simulink model "Pulse_Block"  (R2013b)
settings: Solver=ode3  StartTime=0.0  StopTime=2e-3  FixedStep=sampleTime  MaxStep=MaxStepSize  RelTol=1e-3
undefined symbols (not defined in the file or in its folder): Low, periSam
libraries: dspswit3 x4, simulink x2
settings Model: ExtModeTrigDuration=100  Creator=mainster  LastModifiedBy=mainster
settings OptimizationCC: OptimizeModelRefInitCode=on  LifeSpan=1
settings DebuggingCC: SolverPrmCheckMsg=none
settings HardwareCC: ProdLargestAtomicInteger=Long  ProdLargestAtomicFloat=Double  ProdEndianess=LittleEndian  ProdHWDeviceType=ARM Compatible->ARM Cortex
settings RTWCC: SystemTargetFile=realtime.tlc  GenerateMakefile=off  TemplateMakefile=realtime.tmf  Description=Run on Target Hardware  RTWVerbose=off  ProcessScript=realtime_make_rtw_hook
settings STFCustomTargetCC: TargetLibSuffix=.a  GenerateSampleERTMain=on  ERTCustomFileBanners=on  SupportNonInlinedSFcns=off  SupportVariableSizeSignals=on  MATLABClassNameForMDSCustomization=Simulink.SoftwareTarget.ERTCustomization  GRTInterface=off  SystemTargetFile=realtime.tlc
settings ERTTargetCC: CodeReplacementLibrary=ANSI_C  GenerateSampleERTMain=on  ParMdlRefBuildCompliant=off  CompOptLevelCompliant=off  ConcurrentExecutionCompliant=off  CombineOutputUpdateFcns=off  ERTFirstTimeCompliant=off  SupportContinuousTime=on  SupportVariableSizeSignals=on  ModelStepFunctionPrototypeControlCompliant=off  CPPClassGenCompliant=off  ExtModeMexArgs='192.168.2.111' 0 17725  InlinedParameterPlacement=NonHierarchical  ERTSrcFileBannerTemplate=realtime_code_template.cgt  ERTHdrFileBannerTemplate=realtime_code_template.cgt  ERTDataSrcFileTemplate=realtime_code_template.cgt  ERTDataHdrFileTemplate=realtime_code_template.cgt  ERTCustomFileTemplate=realtime_file_process.tlc

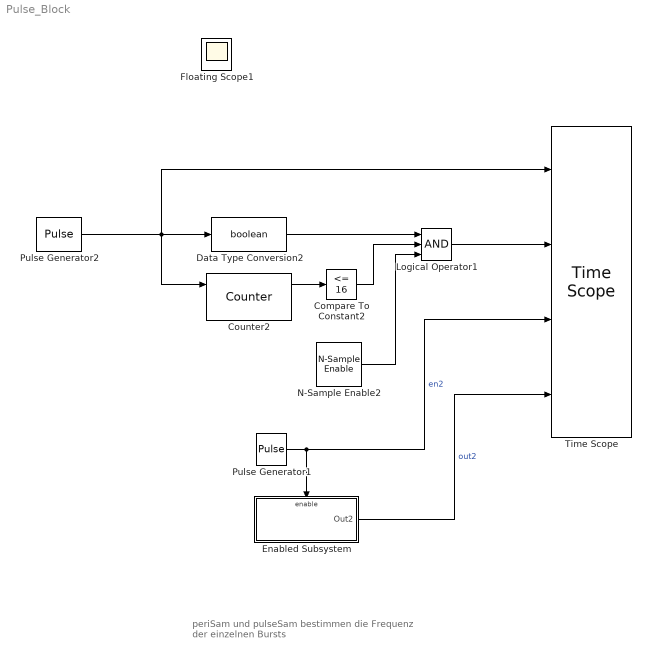
== system Pulse_Block ==
  note: periSam und pulseSam bestimmen die Frequenz
      | der einzelnen Bursts
  Compare To Constant2 : simulink/Logic and Bit Operations/Compare To Constant  relop=<=  const=16  OutDataTypeStr=boolean
  Counter2 : dspswit3/Counter  Direction=Down  CountEvent=Rising edge  CounterSize=User defined  MaxCount=20  InitialCount=0  Output=Count and Hit  HitValue=4  ResetInput=on  SamplesPerFrame=1  Ts=1  CntDtype=double  HitDtype=Logical
  Data Type Conversion2 : DataTypeConversion  OutDataTypeStr=boolean
  Enabled Subsystem : Subsystem  TreatAsAtomicUnit=on
  Logical Operator1 : Logic  Inputs=3  AllPortsSameDT=off  OutDataTypeStr=boolean
  N-Sample Enable2 : dspswit3/N-Sample Enable  N=16*periSam  ActiveLevel=Low (0)  reset=off  TriggerType=Rising edge  Ts=-1  DataType=Logical
  Pulse Generator1 : DiscretePulseGenerator  Period=800  PulseWidth=700  SampleTime=-1
  Pulse Generator2 : DiscretePulseGenerator  Period=periSam  PulseWidth=periSam/2  SampleTime=-1
  Time Scope : TimeScope  NumInputPorts=4  DefaultConfigurationName=spbscopes.TimeScopeBlockCfg
      settings: CopyFcn=scopeextensions.ScopeBlock.onCoreBlockCopy(gcbh);  DeleteFcn=scopeextensions.ScopeBlock.callback(gcbh, 'onBlockDelete');  PreSaveFcn=scopeextensions.ScopeBlock.callback(gcbh, 'onModelSave');  NameChangeFcn=scopeextensions.ScopeBlock.callback(gcbh, 'onBlockRename');  DestroyFcn=scopeextensions.ScopeBlock.onBlockDestroy(gcbh)  CloseFcn=scopeextensions.ScopeBlock.callback(gcbh, 'onBlockClose');  PreDeleteFcn=scopeextensions.ScopeBlock.callback(gcbh, 'onBlockPreDelete');
  Floating Scope1 : Scope
      settings: Floating=on  SaveName=ScopeData3
  wires:
  Enabled Subsystem/1(Out2) -> Time Scope/4  "out2"
  Pulse Generator1/1 -> Enabled Subsystem/Enable, Time Scope/3  "en2"
  Pulse Generator2/1 -> Time Scope/1, Counter2/1, Data Type Conversion2/1
  Data Type Conversion2/1 -> Logical Operator1/1
  Counter2/1 -> Compare To Constant2/1
  Compare To Constant2/1 -> Logical Operator1/2
  N-Sample Enable2/1 -> Logical Operator1/3
  Logical Operator1/1 -> Time Scope/2

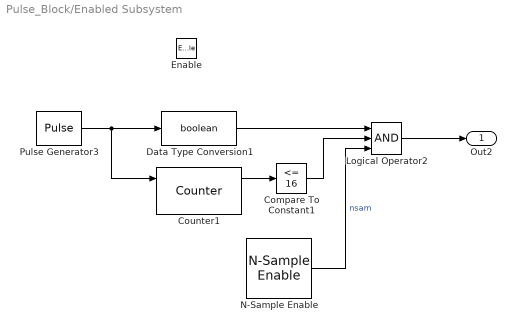
== system Pulse_Block/Enabled Subsystem ==
  Enable : EnablePort  StatesWhenEnabling=reset
  Compare To Constant1 : simulink/Logic and Bit Operations/Compare To Constant  relop=<=  const=16  OutDataTypeStr=boolean
  Counter1 : dspswit3/Counter  Direction=Down  CountEvent=Rising edge  CounterSize=User defined  MaxCount=16  InitialCount=0  Output=Count and Hit  HitValue=4  ResetInput=on  SamplesPerFrame=1  Ts=1  CntDtype=double  HitDtype=Logical
  Data Type Conversion1 : DataTypeConversion  OutDataTypeStr=boolean
  Logical Operator2 : Logic  Inputs=3  AllPortsSameDT=off  OutDataTypeStr=boolean
  N-Sample Enable : dspswit3/N-Sample Enable  N=16*periSam  ActiveLevel=Low (0)  reset=off  TriggerType=Rising edge  Ts=-1  DataType=Logical
  Pulse Generator3 : DiscretePulseGenerator  Period=periSam  PulseWidth=periSam/2  SampleTime=-1
  Out2 : Outport
  wires:
  Pulse Generator3/1 -> Counter1/1, Data Type Conversion1/1
  Data Type Conversion1/1 -> Logical Operator2/1
  Counter1/1 -> Compare To Constant1/1
  Compare To Constant1/1 -> Logical Operator2/2
  Logical Operator2/1 -> Out2/1
  N-Sample Enable/1 -> Logical Operator2/3  "nsam"
